simulink model "PMSM_Drive_custom"  (R2019b)
settings: Solver=VariableStepAuto  StartTime=0.0  StopTime=1  MaxStep=1e-4  RelTol=1e-3
undefined symbols (not defined in the file): kszi0, omega
libraries: simulink x6, PE_components x5, powerlib_meascontrol x3
settings Model: SimulationMode=accelerator  Creator=kissd  LastModifiedBy=kissd

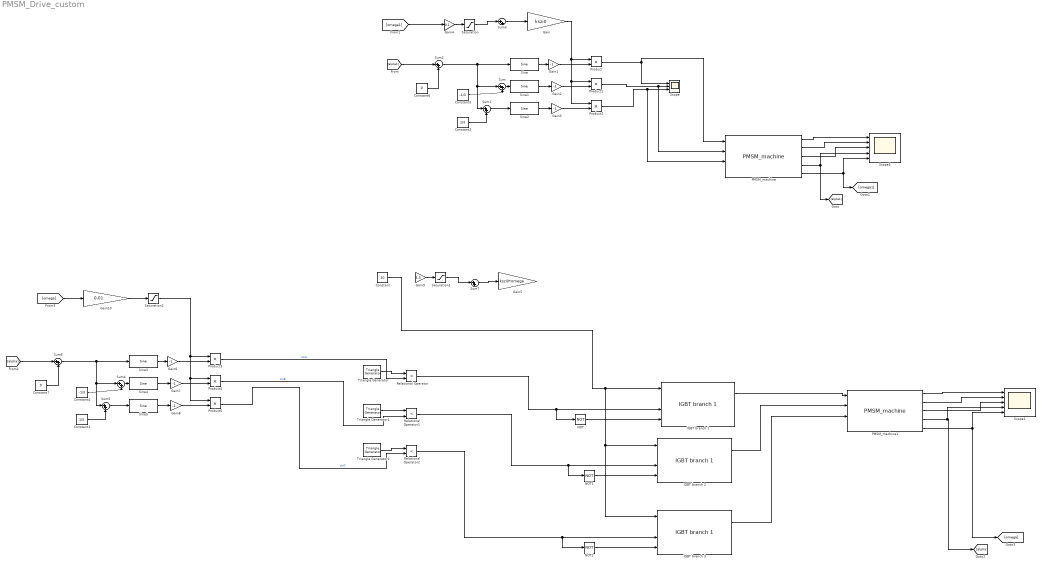
== system PMSM_Drive_custom ==
  Constant : Constant  Value=10
  Constant1 : Constant  Value=1/3
  Constant2 : Constant  Value=1/3
  Constant3 : Constant  Value=-1/3
  Constant4 : Constant  Value=-1/3
  Constant6 : Constant  Value=0
  Constant7 : Constant  Value=0
  Gain : Gain  Gain=kszi0
  Gain{1..3,6..8} (6 alike) : Gain  Gain=-1
  Gain10 : Gain  Gain=0.01
  Gain4 : Gain  Gain=0.1
  Gain5 : Gain  Gain=kszi0*omega
  Gain9 : Gain  Gain=1.5
  IGBT branch 1 : PE_components/IGBT branch 1  SystemSampleTime=-1  Latency=0  AutoFrameSizeCalculation=off
  IGBT branch 2 : PE_components/IGBT branch 1  SystemSampleTime=-1  Latency=0  AutoFrameSizeCalculation=off
  IGBT branch 3 : PE_components/IGBT branch 1  SystemSampleTime=-1  Latency=0  AutoFrameSizeCalculation=off
  NOT : Logic  Operator=NOT  IconShape=distinctive  AllPortsSameDT=off  OutDataTypeStr=boolean
  NOT1 : Logic  Operator=NOT  IconShape=distinctive  AllPortsSameDT=off  OutDataTypeStr=boolean
  NOT2 : Logic  Operator=NOT  IconShape=distinctive  AllPortsSameDT=off  OutDataTypeStr=boolean
  PMSM_machine : PE_components/PMSM_machine  SystemSampleTime=-1  Latency=0  AutoFrameSizeCalculation=off
      link override Gain: Gain=1/Ld
      link override Gain1: Gain=Rs
      link override Gain2: Gain=Rs
      link override Gain4: Gain=1
      link override Gain7: Gain=-3/2
      link override Integrator2: InitialCondition=1
      link override Sum2: Inputs=++-
  PMSM_machine1 : PE_components/PMSM_machine  SystemSampleTime=-1  Latency=0  AutoFrameSizeCalculation=off
      link override Gain1: Gain=Rs
      link override Gain4: Gain=1
      link override Gain7: Gain=-3/2
      link override Integrator2: InitialCondition=1
  Product{,1..5} (6 alike) : Product
  Relational Operator : RelationalOperator  Operator=<  OutDataTypeStr=boolean  RndMeth=Simplest
  Relational Operator1 : RelationalOperator  Operator=<  OutDataTypeStr=boolean  RndMeth=Simplest
  Relational Operator2 : RelationalOperator  Operator=<  OutDataTypeStr=boolean  RndMeth=Simplest
  Saturation : Saturate  UpperLimit=1
  Saturation1 : Saturate  UpperLimit=1.5
  Saturation2 : Saturate  UpperLimit=1
  Scope : Scope  NumInputPorts=3
  Scope1 : Scope  NumInputPorts=5
  Scope5 : Scope  NumInputPorts=5
  Sine{,1..5} (6 alike) : simulink/Lookup Tables/Sine  Formula=sin(2*pi*u)  NumDataPoints=(2^5)+1  OutputWordLength=16  InternalRulePriority=Speed
      settings: SourceProductName=Simulink
  Sum{,1..7} (8 alike) : Sum  Inputs=|++
  Triangle Generator : powerlib_meascontrol/Pulse & Signal Generators/Triangle Generator  Freq=10e3  Phase=90  Ts=0
      settings: SourceProductName=Simscape Electrical
  Triangle Generator1 : powerlib_meascontrol/Pulse & Signal Generators/Triangle Generator  Freq=10e3  Phase=120  Ts=0
      settings: SourceProductName=Simscape Electrical
  Triangle Generator2 : powerlib_meascontrol/Pulse & Signal Generators/Triangle Generator  Freq=10e3  Phase=240  Ts=0
      settings: SourceProductName=Simscape Electrical
  wires:
  PMSM_machine/2 -> Scope5/2
  PMSM_machine/3 -> Scope5/3
  PMSM_machine/1 -> Scope5/1
  Constant/1 -> IGBT branch 1/1, IGBT branch 2/1, IGBT branch 3/1
  Triangle Generator/1 -> Relational Operator/1
  Product3/1 -> Relational Operator/2  "sinA"
  Triangle Generator1/1 -> Relational Operator1/1
  Triangle Generator2/1 -> Relational Operator2/1
  Product5/1 -> Relational Operator2/2  "sinC"
  Relational Operator/1 -> NOT/1, IGBT branch 1/3
  Relational Operator1/1 -> NOT1/1, IGBT branch 2/3
  Relational Operator2/1 -> NOT2/1, IGBT branch 3/3
  PMSM_machine1/2 -> Scope1/2
  PMSM_machine1/3 -> Scope1/3
  PMSM_machine1/1 -> Scope1/1
  IGBT branch 3/1 -> PMSM_machine1/3
  IGBT branch 1/1 -> PMSM_machine1/1
  IGBT branch 2/1 -> PMSM_machine1/2
  NOT/1 -> IGBT branch 1/4
  NOT1/1 -> IGBT branch 2/4
  NOT2/1 -> IGBT branch 3/4
  PMSM_machine/4 -> [alpha1], Scope5/4
  PMSM_machine/5 -> [omega1], Scope5/5
  Sum/1 -> Sine1/1
  Sum1/1 -> Sine2/1
  Constant3/1 -> Sum/2
  Constant2/1 -> Sum1/2
  Sine/1 -> Gain1/1
  Sine1/1 -> Gain2/1
  Sine2/1 -> Gain3/1
  Product1/1 -> PMSM_machine/2, Scope/2
  Product/1 -> Scope/1, PMSM_machine/1
  Product2/1 -> PMSM_machine/3, Scope/3
  Gain/1 -> Product2/1, Product1/1, Product/1
  [alpha1] -> Sum2/1
  Sum2/1 -> Sum1/1, Sum/1, Sine/1
  Constant6/1 -> Sum2/2
  Sum3/1 -> Gain/1
  Gain4/1 -> Saturation/1
  Gain1/1 -> Product/2
  Gain2/1 -> Product1/2
  Gain3/1 -> Product2/2
  [omega1] -> Gain4/1
  Saturation/1 -> Sum3/1
  Sum6/1 -> Sum5/1, Sum4/1, Sine3/1
  Sum4/1 -> Sine4/1
  Sine3/1 -> Gain6/1
  Sine4/1 -> Gain7/1
  Sum5/1 -> Sine5/1
  Sine5/1 -> Gain8/1
  Constant4/1 -> Sum4/2
  Constant1/1 -> Sum5/2
  Gain7/1 -> Product4/2
  Constant7/1 -> Sum6/2
  [alpha] -> Sum6/1
  Gain8/1 -> Product5/2
  Gain6/1 -> Product3/2
  Product4/1 -> Relational Operator1/2  "sinB"
  PMSM_machine1/5 -> Scope1/5, [omega]
  PMSM_machine1/4 -> Scope1/4, [alpha]
  Gain9/1 -> Saturation1/1
  Saturation1/1 -> Sum7/1
  Sum7/1 -> Gain5/1
  [omega] -> Gain10/1
  Gain10/1 -> Saturation2/1
  Saturation2/1 -> Product5/1, Product4/1, Product3/1
